simulink model "freefalling"  (R2017a)
settings: Solver=FixedStepAuto  StartTime=0.0  StopTime=10.0  FixedStep=0.001  RelTol=1e-3
undefined symbols (not defined in the file): c, d, df, g, m
settings Model: Creator=22132  LastModifiedBy=22132

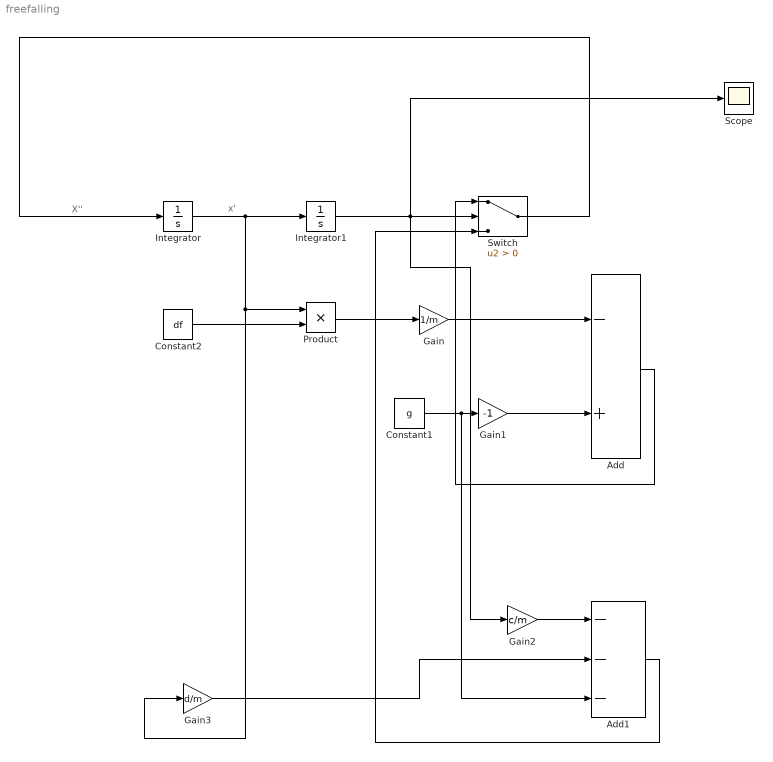
== system freefalling ==
  note: x'
  note: X''
  Add : Sum  Inputs=-+
  Add1 : Sum  Inputs=---
  Constant1 : Constant  Value=g
  Constant2 : Constant  Value=df
  Gain : Gain  Gain=1/m
  Gain1 : Gain  Gain=-1
  Gain2 : Gain  Gain=c/m
  Gain3 : Gain  Gain=d/m
  Integrator : Integrator
  Integrator1 : Integrator  InitialCondition=1
  Product : Product
  Scope : Scope
  Switch : Switch  Criteria=u2 > Threshold
  wires:
  Integrator/1 -> Gain3/1, Product/1, Integrator1/1
  Constant2/1 -> Product/2
  Product/1 -> Gain/1
  Gain/1 -> Add/1
  Constant1/1 -> Add1/3, Gain1/1
  Gain1/1 -> Add/2
  Integrator1/1 -> Gain2/1, Scope/1, Switch/2
  Switch/1 -> Integrator/1
  Add/1 -> Switch/1
  Add1/1 -> Switch/3
  Gain3/1 -> Add1/2
  Gain2/1 -> Add1/1
